simulink model "BPSK_Rayleigh_FLAT_FLAT_exercise"  (R2021b)
settings: Solver=VariableStepAuto  StartTime=0.0  StopTime=Inf  RelTol=1e-3
undefined symbols (not defined in the file or in its folder): gaussian
libraries: simulink x12, commdigbbndpm3 x8, commchan3 x6, commrandsrc3 x6, commsink2 x6, commdigbbndam3 x4
settings Model: Creator=roberto  LastModifiedBy=Omar

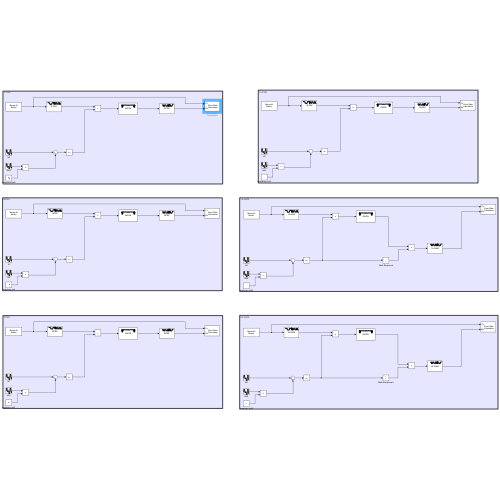
[thumbnail: Simulink's stored preview of the top-level diagram]
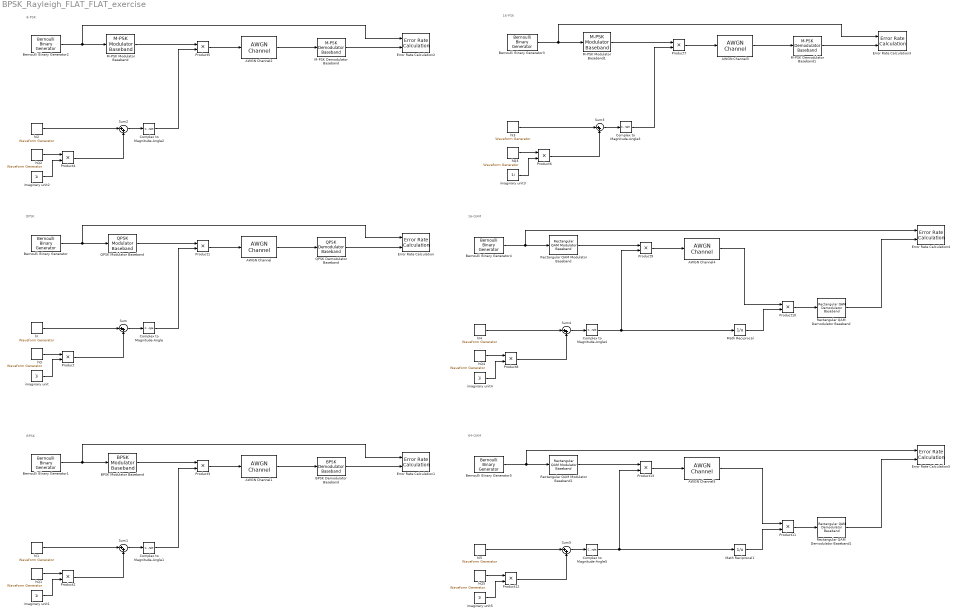
== system BPSK_Rayleigh_FLAT_FLAT_exercise ==
  note: 64-QAM
  note: 16-QAM
  note: 16-PSK
  note: 8-PSK
  note: BPSK
  note: QPSK
  AWGN Channel{,1..5} (6 alike) : commchan3/AWGN Channel  InputProcessing=Columns as channels (frame based)  seed=67  noiseMode="Signal to noise ratio  (Eb/No)"  EbNodB=EbNo  EsNodB=10  SNRdB=10  bitsPerSym=1  Ps=1  Tsym=1  variance=1
  BPSK Demodulator Baseband : commdigbbndpm3/BPSK Demodulator Baseband  DecType=Hard decision  VarSource=Dialog  Variance=1  Ph=0  outDtype=Inherit via internal rule  derotateFactorWordLen=16  derotateFactorDataTypeStr=Inherit: Same word length as input  derotateFactorLastDataTypeStr=Inherit: Same word length as input
  BPSK Modulator Baseband : commdigbbndpm3/BPSK Modulator Baseband  Ph=0  outDtype=double  outWordLen=16  outUDDataType=sfix(16)  outFracLenMode=Best precision  outFracLen=15  outDataTypeStr=double  outLastDataTypeStr=double
  Bernoulli Binary Generator{,1..5} (6 alike) : commrandsrc3/Bernoulli Binary Generator  ProbabilityOfZero=0.5  SeedSource=Auto  Seed=0  SampleTime=1  SamplesPerFrame=1  OutputDataType=double  SimulateUsing=Interpreted execution
  Complex to Magnitude-Angle{,1..5} (6 alike) : ComplexToMagnitudeAngle  Output=Magnitude
  Error Rate Calculation : commsink2/Error Rate Calculation  N=0  st_delay=0  cp_mode=Entire frame  subframe=[]  PMode=Workspace  WsName=ErrorVec0  RsMode2=off  stop=on  numErr=maxNumErrs  maxBits=maxNumBits
  Error Rate Calculation1 : commsink2/Error Rate Calculation  N=0  st_delay=0  cp_mode=Entire frame  subframe=[]  PMode=Workspace  WsName=ErrorVec  RsMode2=off  stop=on  numErr=maxNumErrs  maxBits=maxNumBits
  Error Rate Calculation2 : commsink2/Error Rate Calculation  N=0  st_delay=0  cp_mode=Entire frame  subframe=[]  PMode=Workspace  WsName=ErrorVec1  RsMode2=off  stop=on  numErr=maxNumErrs  maxBits=maxNumBits
  Error Rate Calculation3 : commsink2/Error Rate Calculation  N=0  st_delay=0  cp_mode=Entire frame  subframe=[]  PMode=Workspace  WsName=ErrorVec2  RsMode2=off  stop=on  numErr=maxNumErrs  maxBits=maxNumBits
  Error Rate Calculation4 : commsink2/Error Rate Calculation  N=0  st_delay=0  cp_mode=Entire frame  subframe=[]  PMode=Workspace  WsName=ErrorVec3  RsMode2=off  stop=on  numErr=maxNumErrs  maxBits=maxNumBits
  Error Rate Calculation5 : commsink2/Error Rate Calculation  N=0  st_delay=0  cp_mode=Entire frame  subframe=[]  PMode=Workspace  WsName=ErrorVec4  RsMode2=off  stop=on  numErr=maxNumErrs  maxBits=maxNumBits
  M-PSK Demodulator Baseband : commdigbbndpm3/M-PSK Demodulator Baseband  M=8  OutType=Integer  DecType=Hard decision  VarSource=Dialog  Variance=1  Dec=Gray  Mapping=[0:7]  Ph=pi/8  outDtype1=Inherit via internal rule  outDtype2=Inherit via internal rule  derotateFactorWordLen=16  derotateFactorDataTypeStr=Inherit: Same word length as input  derotateFactorLastDataTypeStr=Inherit: Same word length as input
  M-PSK Demodulator Baseband1 : commdigbbndpm3/M-PSK Demodulator Baseband  M=16  OutType=Integer  DecType=Hard decision  VarSource=Dialog  Variance=1  Dec=Gray  Mapping=[0:7]  Ph=pi/8  outDtype1=Inherit via internal rule  outDtype2=Inherit via internal rule  derotateFactorWordLen=16  derotateFactorDataTypeStr=Inherit: Same word length as input  derotateFactorLastDataTypeStr=Inherit: Same word length as input
  M-PSK Modulator Baseband : commdigbbndpm3/M-PSK Modulator Baseband  M=8  InType=Integer  Enc=Gray  Mapping=[0:7]  Ph=pi/8  outDtype=double  outWordLen=16  outUDDataType=sfix(16)  outFracLenMode=Best precision  outFracLen=15  outDataTypeStr=double  outLastDataTypeStr=double
  M-PSK Modulator Baseband1 : commdigbbndpm3/M-PSK Modulator Baseband  M=16  InType=Integer  Enc=Gray  Mapping=[0:7]  Ph=pi/8  outDtype=double  outWordLen=16  outUDDataType=sfix(16)  outFracLenMode=Best precision  outFracLen=15  outDataTypeStr=double  outLastDataTypeStr=double
  Math Reciprocal : Math  Operator=reciprocal  SignedPower=on  SaturateOnIntegerOverflow=on
  Math Reciprocal1 : Math  Operator=reciprocal  SignedPower=on  SaturateOnIntegerOverflow=on
  Product{,1..13} (14 alike) : Product
  QPSK Demodulator Baseband : commdigbbndpm3/QPSK Demodulator Baseband  OutType=Integer  DecType=Hard decision  VarSource=Dialog  Variance=1  Dec=Gray  Ph=pi/4  outDtype1=Inherit via internal rule  outDtype2=Inherit via internal rule  derotateFactorWordLen=16  derotateFactorDataTypeStr=Inherit: Same word length as input  derotateFactorLastDataTypeStr=Inherit: Same word length as input
  QPSK Modulator Baseband : commdigbbndpm3/QPSK Modulator Baseband  InType=Integer  Enc=Gray  Ph=pi/4  outDtype=double  outWordLen=16  outUDDataType=sfix(16)  outFracLenMode=Best precision  outFracLen=15  outDataTypeStr=double  outLastDataTypeStr=double
  Rectangular QAM Demodulator Baseband : commdigbbndam3/Rectangular QAM Demodulator Baseband  M=16  OutType=Integer  DecType=Hard decision  VarSource=Dialog  Variance=1  Dec=Gray  Mapping=[0:15]  PowType=Min. distance between symbols  MinDist=2  AvgPow=1  PeakPow=1  Ph=0  outDtype1=Inherit via internal rule  outDtype2=Inherit via internal rule  derotateFactorWordLen=16  derotateFactorDataTypeStr=Inherit: Same word length as input  derotateFactorLastDataTypeStr=Inherit: Same word length as input  denormFactorWordLen=16  denormFactorDataTypeStr=Inherit: Same word length as input  denormFactorLastDataTypeStr=Inherit: Same word length as input  prodOutWordLen=32  prodOutOverflowMode=Wrap  prodOutRoundingMode=Floor  prodOutOvFlMode=off  prodOutOvFlModeLastStrValue=off  sumWordLen=32
  Rectangular QAM Demodulator Baseband1 : commdigbbndam3/Rectangular QAM Demodulator Baseband  M=64  OutType=Integer  DecType=Hard decision  VarSource=Dialog  Variance=1  Dec=Gray  Mapping=[0:15]  PowType=Min. distance between symbols  MinDist=2  AvgPow=1  PeakPow=1  Ph=0  outDtype1=Inherit via internal rule  outDtype2=Inherit via internal rule  derotateFactorWordLen=16  derotateFactorDataTypeStr=Inherit: Same word length as input  derotateFactorLastDataTypeStr=Inherit: Same word length as input  denormFactorWordLen=16  denormFactorDataTypeStr=Inherit: Same word length as input  denormFactorLastDataTypeStr=Inherit: Same word length as input  prodOutWordLen=32  prodOutOverflowMode=Wrap  prodOutRoundingMode=Floor  prodOutOvFlMode=off  prodOutOvFlModeLastStrValue=off  sumWordLen=32
  Rectangular QAM Modulator Baseband : commdigbbndam3/Rectangular QAM Modulator Baseband  M=16  InType=Integer  Enc=Gray  Mapping=[0:15]  PowType=Min. distance between symbols  MinDist=2  AvgPow=1  PeakPow=1  Ph=0  outDtype=double  outWordLen=16  outUDDataType=sfix(16)  outFracLenMode=Best precision  outFracLen=15  outDataTypeStr=double  outLastDataTypeStr=double
  Rectangular QAM Modulator Baseband1 : commdigbbndam3/Rectangular QAM Modulator Baseband  M=64  InType=Integer  Enc=Gray  Mapping=[0:15]  PowType=Min. distance between symbols  MinDist=2  AvgPow=1  PeakPow=1  Ph=0  outDtype=double  outWordLen=16  outUDDataType=sfix(16)  outFracLenMode=Best precision  outFracLen=15  outDataTypeStr=double  outLastDataTypeStr=double
  Sum{,1..5} (6 alike) : Sum  Inputs=|++
  hI{,1..5} (6 alike) : simulink/Sources/Waveform Generator  OutMin=[]  OutMax=[]  OutDataTypeStr=double  SelectedSignal=1  Signals=gaussian('Mean',0,'Variance',0.5,'Seed',1)  BlockNames=MultiportSwitch_fb556a3493b141a  SampleTime=1
  hQ{,1..5} (6 alike) : simulink/Sources/Waveform Generator  OutMin=[]  OutMax=[]  OutDataTypeStr=double  SelectedSignal=1  Signals=gaussian('Mean',0,'Variance',0.5,'Seed',67)  BlockNames=MultiportSwitch_47572b58e7994c6  SampleTime=1
  imaginary unit{,1..5} (6 alike) : Constant  Value=1i
  wires:
  QPSK Demodulator Baseband/1 -> Error Rate Calculation/2
  QPSK Modulator Baseband/1 -> Product1/1
  hI/1 -> Sum/1
  Sum/1 -> Complex to Magnitude-Angle/1
  Bernoulli Binary Generator/1 -> QPSK Modulator Baseband/1, Error Rate Calculation/1
  AWGN Channel/1 -> QPSK Demodulator Baseband/1
  imaginary unit/1 -> Product/2
  Product/1 -> Sum/2
  Product1/1 -> AWGN Channel/1
  Complex to Magnitude-Angle/1 -> Product1/2
  hQ/1 -> Product/1
  hQ1/1 -> Product2/1
  Product3/1 -> AWGN Channel1/1
  imaginary unit1/1 -> Product2/2
  Sum1/1 -> Complex to Magnitude-Angle1/1
  Bernoulli Binary Generator1/1 -> Error Rate Calculation1/1, BPSK Modulator Baseband/1
  BPSK Modulator Baseband/1 -> Product3/1
  BPSK Demodulator Baseband/1 -> Error Rate Calculation1/2
  Complex to Magnitude-Angle1/1 -> Product3/2
  AWGN Channel1/1 -> BPSK Demodulator Baseband/1
  Product2/1 -> Sum1/2
  hI1/1 -> Sum1/1
  AWGN Channel2/1 -> M-PSK Demodulator Baseband/1
  M-PSK Demodulator Baseband/1 -> Error Rate Calculation2/2
  Product4/1 -> Sum2/2
  Product5/1 -> AWGN Channel2/1
  M-PSK Modulator Baseband/1 -> Product5/1
  imaginary unit2/1 -> Product4/2
  Complex to Magnitude-Angle2/1 -> Product5/2
  hQ2/1 -> Product4/1
  hI2/1 -> Sum2/1
  Bernoulli Binary Generator2/1 -> M-PSK Modulator Baseband/1, Error Rate Calculation2/1
  Sum2/1 -> Complex to Magnitude-Angle2/1
  Bernoulli Binary Generator3/1 -> M-PSK Modulator Baseband1/1, Error Rate Calculation3/1
  Product6/1 -> Sum3/2
  Sum3/1 -> Complex to Magnitude-Angle3/1
  Product7/1 -> AWGN Channel3/1
  Complex to Magnitude-Angle3/1 -> Product7/2
  hI3/1 -> Sum3/1
  hQ3/1 -> Product6/1
  AWGN Channel3/1 -> M-PSK Demodulator Baseband1/1
  imaginary unit3/1 -> Product6/2
  M-PSK Modulator Baseband1/1 -> Product7/1
  M-PSK Demodulator Baseband1/1 -> Error Rate Calculation3/2
  Product10/1 -> Rectangular QAM Demodulator Baseband/1
  Math Reciprocal/1 -> Product10/2
  Rectangular QAM Demodulator Baseband/1 -> Error Rate Calculation4/2
  Rectangular QAM Modulator Baseband/1 -> Product9/1
  Product9/1 -> AWGN Channel4/1
  Complex to Magnitude-Angle4/1 -> Math Reciprocal/1, Product9/2
  AWGN Channel4/1 -> Product10/1
  Product8/1 -> Sum4/2
  Bernoulli Binary Generator4/1 -> Rectangular QAM Modulator Baseband/1, Error Rate Calculation4/1
  Sum4/1 -> Complex to Magnitude-Angle4/1
  hI4/1 -> Sum4/1
  hQ4/1 -> Product8/1
  imaginary unit4/1 -> Product8/2
  Rectangular QAM Demodulator Baseband1/1 -> Error Rate Calculation5/2
  AWGN Channel5/1 -> Product11/1
  Product12/1 -> Sum5/2
  Product13/1 -> AWGN Channel5/1
  imaginary unit5/1 -> Product12/2
  Rectangular QAM Modulator Baseband1/1 -> Product13/1
  Bernoulli Binary Generator5/1 -> Error Rate Calculation5/1, Rectangular QAM Modulator Baseband1/1
  hQ5/1 -> Product12/1
  Sum5/1 -> Complex to Magnitude-Angle5/1
  Complex to Magnitude-Angle5/1 -> Product13/2, Math Reciprocal1/1
  Math Reciprocal1/1 -> Product11/2
  Product11/1 -> Rectangular QAM Demodulator Baseband1/1
  hI5/1 -> Sum5/1
